simulink model "sim_msd_i_pd_cont_R2015a"  (R2015a)
settings: Solver=ode4  SolverMode=SingleTasking  StartTime=0.0  StopTime=9  FixedStep=0.001  RelTol=1e-3
values from neighbouring files (symbols this model uses):
  kD = sol2.kD    [example_06_02a_sym.m]    (also in example_06_02b.m = (2*zeta_m*wm - a1)/b0; example_06_02b_sym.m; example_06_03.m = 1; example_06_04.m = 1)
  kI = 6    [example_06_04.m]    (also in example_06_04_R2015a.m; example_06_04_R2018a.m; example_06_06a1.m = 0.8; example_06_06a2.m = 1.2)
  kP = (wm^2 - a0)/b0    [example_06_01.m]    (also in example_06_02a.m = 4; example_06_02a_sym.m = sol2.kP; example_06_02b.m = 6.8; example_06_02b_sym.m = sol2.kP)
settings Model: CovMetricSettings=dwe  CovHtmlReporting=off  covSaveCumulativeToWorkspaceVar=off  CovSaveSingleToWorkspaceVar=off  CovExternalEMLEnable=on  Creator=kawata  LastModifiedBy=kawata
settings DataIOCC: LimitDataPoints=off  SaveFormat=Dataset
settings DebuggingCC: SFUnexpectedBacktrackingDiag=error  SFNoUnconditionalDefaultTransitionDiag=error
settings HardwareCC: ProdBitPerPointer=64  ProdLargestAtomicFloat=Float  ProdIntDivRoundTo=Zero  ProdEndianess=LittleEndian  ProdHWDeviceType=Specified
settings ModelReferenceCC: PropagateSignalLabelsOutOfModel=on
settings SFSimCC: SimUseLocalCustomCode=on
settings RTWCC: RTWUseLocalCustomCode=on
settings GRTTargetCC: TargetLangStandard=C99 (ISO)  GeneratePreprocessorConditionals=Use local settings

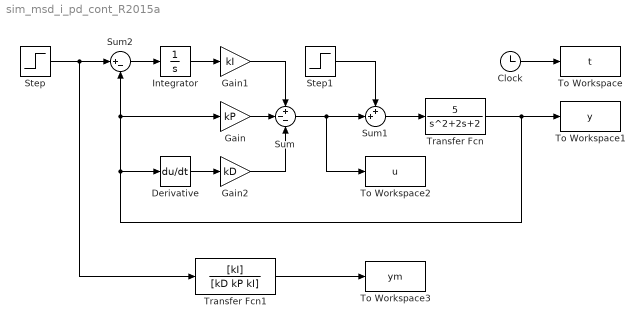
== system sim_msd_i_pd_cont_R2015a ==
  Clock : Clock
  Derivative : Derivative
  Gain : Gain  Gain=kP
  Gain1 : Gain  Gain=kI
  Gain2 : Gain  Gain=kD
  Integrator : Integrator
  Step : Step  SampleTime=0
  Step1 : Step  Time=5  SampleTime=0
  Sum : Sum  Inputs=+--
  Sum1 : Sum  Inputs=++|
  Sum2 : Sum  Inputs=|+-
  To Workspace : ToWorkspace  VariableName=t  SampleTime=-1
  To Workspace1 : ToWorkspace  VariableName=y  SampleTime=-1
  To Workspace2 : ToWorkspace  VariableName=u  SampleTime=-1
  To Workspace3 : ToWorkspace  VariableName=ym  SampleTime=-1
  Transfer Fcn : TransferFcn  Numerator=[5]  Denominator=[1 2 2]
  Transfer Fcn1 : TransferFcn  Numerator=[kI]  Denominator=[kD kP kI]
  wires:
  Gain1/1 -> Sum/1
  Gain/1 -> Sum/2
  Gain2/1 -> Sum/3
  Sum/1 -> To Workspace2/1, Sum1/2
  Sum1/1 -> Transfer Fcn/1
  Transfer Fcn/1 -> To Workspace1/1, Gain/1, Sum2/2, Derivative/1
  Integrator/1 -> Gain1/1
  Derivative/1 -> Gain2/1
  Step/1 -> Transfer Fcn1/1, Sum2/1
  Step1/1 -> Sum1/1
  Clock/1 -> To Workspace/1
  Sum2/1 -> Integrator/1
  Transfer Fcn1/1 -> To Workspace3/1
